simulink model "swerve_chassis"  (R2025b)
settings: Solver=VariableStepAuto  StartTime=0.0  StopTime=20  RelTol=1e-2  AbsTol=1e-3
undefined symbols (not defined in the file): X, Y, Z
libraries: sm_lib x35, nesl_utility x18, slpidlib x8
(part 2 of 2)

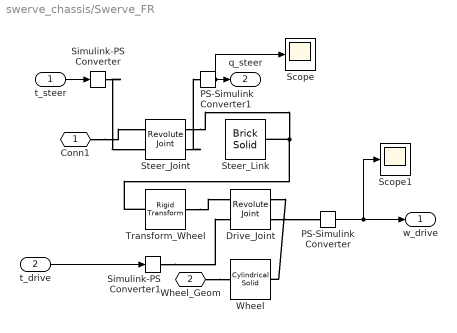
== system swerve_chassis/Swerve_FR ==
  t_steer : Inport
  t_drive : Inport  Port=2
  Drive_Joint : sm_lib/Joints/Revolute Joint  JointMode=Normal  CompositeWrenchDir=FollowerOnBase  CompositeWrenchFrame=BaseFrame  SenseConstraintForce=off  SenseConstraintTorque=off  SenseTotalForce=off  SenseTotalTorque=off  PositionTargetSpecify=off  PositionTargetPriority=High  PositionTargetValue=0  PositionTargetValueUnits=deg  VelocityTargetSpecify=off  VelocityTargetPriority=High  VelocityTargetValue=0  VelocityTargetValueUnits=deg/s  EquilibriumPosition=0  EquilibriumPositionUnits=deg  SpringStiffness=0  SpringStiffnessUnits=N*m/deg  DampingCoefficient=0  DampingCoefficientUnits=N*m/(deg/s)  LowerLimitSpecify=off  LowerLimitBound=-90  LowerLimitBoundUnits=deg  LowerLimitStiffness=1e4  LowerLimitStiffnessUnits=N*m/deg  LowerLimitDamping=10  LowerLimitDampingUnits=N*m/(deg/s)  LowerLimitTransitionRegionWidth=0.1  LowerLimitTransitionRegionWidthUnits=deg  UpperLimitSpecify=off  UpperLimitBound=90  UpperLimitBoundUnits=deg  UpperLimitStiffness=1e4  UpperLimitStiffnessUnits=N*m/deg  UpperLimitDamping=10  UpperLimitDampingUnits=N*m/(deg/s)  UpperLimitTransitionRegionWidth=0.1  UpperLimitTransitionRegionWidthUnits=deg  TorqueActuationMode=InputTorque  MotionActuationMode=ComputedMotion  SensePosition=off  SenseVelocity=on  SenseAcceleration=off  SenseTorqueForce=off  SenseLowerLimitTorqueForce=off  SenseUpperLimitTorqueForce=off
  PS-Simulink Converter : nesl_utility/PS-Simulink Converter  PhysicalDomain=network_engine_domain  SubClassName=ps_output  LeftPortType=input  RightPortType=output  PseudoPeriodic=off  Frequencies=[]  VectorFormat=inherit  Unit=rad/s  AffineConversion=off
  PS-Simulink Converter1 : nesl_utility/PS-Simulink Converter  PhysicalDomain=network_engine_domain  SubClassName=ps_output  LeftPortType=input  RightPortType=output  PseudoPeriodic=off  Frequencies=[]  VectorFormat=inherit  Unit=rad  AffineConversion=off
  Scope : Scope
      settings: ActiveDisplayYMinimum=-1  ActiveDisplayYMaximum=1  DataLoggingVariableName=ScopeData2
  Scope1 : Scope
      settings: ActiveDisplayYMinimum=-1  ActiveDisplayYMaximum=1  DataLoggingVariableName=ScopeData3
  Simulink-PS Converter : nesl_utility/Simulink-PS Converter  PhysicalDomain=network_engine_domain  SubClassName=ps_input  LeftPortType=input  RightPortType=output  PseudoPeriodic=off  Frequencies=[]  NoiseDistribution=none  NoiseParameters=[]  Unit=1  AffineConversion=off  FilteringAndDerivatives=provide  SimscapeFilterOrder=1  InputFilterTimeConstant=0.001  UdotUserProvided=0
  Simulink-PS Converter1 : nesl_utility/Simulink-PS Converter  PhysicalDomain=network_engine_domain  SubClassName=ps_input  LeftPortType=input  RightPortType=output  PseudoPeriodic=off  Frequencies=[]  NoiseDistribution=none  NoiseParameters=[]  Unit=1  AffineConversion=off  FilteringAndDerivatives=provide  SimscapeFilterOrder=1  InputFilterTimeConstant=0.001  UdotUserProvided=0
  Steer_Joint : sm_lib/Joints/Revolute Joint  JointMode=Normal  CompositeWrenchDir=FollowerOnBase  CompositeWrenchFrame=BaseFrame  SenseConstraintForce=off  SenseConstraintTorque=off  SenseTotalForce=off  SenseTotalTorque=off  PositionTargetSpecify=off  PositionTargetPriority=High  PositionTargetValue=0  PositionTargetValueUnits=deg  VelocityTargetSpecify=off  VelocityTargetPriority=High  VelocityTargetValue=0  VelocityTargetValueUnits=deg/s  EquilibriumPosition=0  EquilibriumPositionUnits=deg  SpringStiffness=0  SpringStiffnessUnits=N*m/deg  DampingCoefficient=0  DampingCoefficientUnits=N*m/(deg/s)  LowerLimitSpecify=off  LowerLimitBound=-90  LowerLimitBoundUnits=deg  LowerLimitStiffness=1e4  LowerLimitStiffnessUnits=N*m/deg  LowerLimitDamping=10  LowerLimitDampingUnits=N*m/(deg/s)  LowerLimitTransitionRegionWidth=0.1  LowerLimitTransitionRegionWidthUnits=deg  UpperLimitSpecify=off  UpperLimitBound=90  UpperLimitBoundUnits=deg  UpperLimitStiffness=1e4  UpperLimitStiffnessUnits=N*m/deg  UpperLimitDamping=10  UpperLimitDampingUnits=N*m/(deg/s)  UpperLimitTransitionRegionWidth=0.1  UpperLimitTransitionRegionWidthUnits=deg  TorqueActuationMode=InputTorque  MotionActuationMode=ComputedMotion  SensePosition=on  SenseVelocity=off  SenseAcceleration=off  SenseTorqueForce=off  SenseLowerLimitTorqueForce=off  SenseUpperLimitTorqueForce=off
  Steer_Link : sm_lib/Body Elements/Brick Solid  BrickDimensions=[0.05 0.05 0.1]  BrickDimensionsUnits=m  ExportEntireGeometry=off  InertiaType=Custom  BasedOnType=Density  Density=1000  DensityUnits=kg/m^3  Mass=1  MassUnits=kg  CenterOfMass=[0 0 0]  CenterOfMassUnits=m  MomentsOfInertia=[1 1 1]  MomentsOfInertiaUnits=kg*m^2  ProductsOfInertia=[0 0 0]  ProductsOfInertiaUnits=kg*m^2  GraphicType=FromGeometry  MarkerShape=Sphere  MarkerSize=10  GraphicVisPropType=SimpleVisualProperties  GraphicDiffuseColor=[1 1 0]  GraphicOpacity=1  GraphicSpecularColor=[0.5 0.5 0.5 1.0]  GraphicAmbientColor=[0.15 0.15 0.15 1.0]  GraphicEmissiveColor=[0.0 0.0 0.0 1.0]  GraphicShininess=75  DoExposeReferenceFrame=on  SerializedFrames=<Frames/>
  Transform_Wheel : sm_lib/Frames and Transforms/Rigid Transform  RotationMethod=StandardAxis  FollAlignAxisA=+X  BaseAlignAxisA=+Y  FollAlignAxisB=+Y  BaseAlignAxisB=+Z  RotationStandardAxis=+X  RotationAngle=90  RotationAngleUnits=deg  RotationArbitraryAxis=[0 0 1]  RotationSequenceAxes=FollowerAxes  RotationSequence=XYX  RotationSequenceAngles=[0 0 0]  RotationSequenceAnglesUnits=deg  RotationMatrix=[1 0 0;0 1 0;0 0 1]  Quaternion=[1 0 0 0]  TranslationMethod=StandardAxis  TranslationCartesianOffset=[0 0 0]  TranslationCartesianOffsetUnits=m  TranslationStandardAxis=-Z  TranslationStandardOffset=0.05  TranslationStandardOffsetUnits=m  TranslationROffset=0  TranslationROffsetUnits=m  TranslationThetaOffset=0  TranslationThetaOffsetUnits=deg  TranslationZOffset=0  TranslationZOffsetUnits=m
  Wheel : sm_lib/Body Elements/Cylindrical Solid  CylinderRadius=0.05  CylinderRadiusUnits=m  CylinderLength=0.03  CylinderLengthUnits=m  ExportEntireGeometry=on  InertiaType=Custom  BasedOnType=Density  Density=1000  DensityUnits=kg/m^3  Mass=1  MassUnits=kg  CenterOfMass=[0 0 0]  CenterOfMassUnits=m  MomentsOfInertia=[1 1 1]  MomentsOfInertiaUnits=kg*m^2  ProductsOfInertia=[0 0 0]  ProductsOfInertiaUnits=kg*m^2  GraphicType=FromGeometry  MarkerShape=Sphere  MarkerSize=10  GraphicVisPropType=AdvancedVisualProperties  GraphicDiffuseColor=[1 0 0]  GraphicOpacity=1  GraphicSpecularColor=[0.5 0.5 0.5 1.0]  GraphicAmbientColor=[0.15 0.15 0.15 1.0]  GraphicEmissiveColor=[0.0 0.0 0.0 1.0]  GraphicShininess=75  DoExposeReferenceFrame=on  SerializedFrames=<Frames/>
  Conn1 : PMIOPort  Side=Left
  Wheel_Geom : PMIOPort  Port=2  Side=Left
  w_drive : Outport
  q_steer : Outport  Port=2
  wires:
  t_steer/1 -> Simulink-PS Converter/1
  PS-Simulink Converter1/1 -> Scope/1, q_steer/1
  t_drive/1 -> Simulink-PS Converter1/1
  PS-Simulink Converter/1 -> Scope1/1, w_drive/1
  connections:
  Conn1/RConn1 -- Steer_Joint/LConn1
  Steer_Joint/RConn1 -- Transform_Wheel/LConn1 -- Steer_Link/RConn1
  Transform_Wheel/RConn1 -- Drive_Joint/LConn1
  Drive_Joint/RConn1 -- Wheel/RConn1
  Wheel_Geom/RConn1 -- Wheel/LConn1
  Simulink-PS Converter/RConn1 -- Steer_Joint/LConn2
  Simulink-PS Converter1/RConn1 -- Drive_Joint/LConn2
  Drive_Joint/RConn2 -- PS-Simulink Converter/LConn1
  Steer_Joint/RConn2 -- PS-Simulink Converter1/LConn1

== matlab function swerve_chassis/MATLAB Function1 ==
  data: vx input; FL_Angle output; FL_Vel output; vy input; omega input; FR_Angle output; FR_Vel output; BL_Angle output; BL_Vel output; BR_Angle output; BR_Vel output
function [FL_Angle, FL_Vel, FR_Angle, FR_Vel, BL_Angle, BL_Vel, BR_Angle, BR_Vel] = IK_fcn(vx, vy, omega)
    % --- 尺寸参数 ---
    L = 0.5;  % 车长 (影响 Y 轴分量)
    W = 0.5;  % 车宽 (影响 X 轴分量)
    R = 0.05; % 车轮半径 (米)
    
    % --- 1. 绝对纯净的数学速度分量 (修复了 L 和 W 的交叉对应) ---
    FL_vx = vx - omega * (W / 2);
    FL_vy = vy + omega * (L / 2);
    
    FR_vx = vx + omega * (W / 2);
    FR_vy = vy + omega * (L / 2);
    
    BL_vx = vx - omega * (W / 2);
    BL_vy = vy - omega * (L / 2);
    
    BR_vx = vx + omega * (W / 2);
    BR_vy = vy - omega * (L / 2);

    % --- 2. 角度对齐 ---
    % 因为你已经在 Simscape 硬件的三维模型里加了 180 度，这里必须是 0
    offset = 0; 
    
    FL_Angle = atan2(FL_vy, FL_vx) + offset;
    FR_Angle = atan2(FR_vy, FR_vx) + offset;
    BL_Angle = atan2(BL_vy, BL_vx) + offset;
    BR_Angle = atan2(BR_vy, BR_vx) + offset;

    % --- 3. 速度输出转换 (直接除以车轮半径 R，将 m/s 转换为 rad/s) ---
    FL_Vel = sqrt(FL_vx^2 + FL_vy^2) / R;
    BL_Vel = sqrt(BL_vx^2 + BL_vy^2) / R;
    FR_Vel = sqrt(FR_vx^2 + FR_vy^2) / R; 
    BR_Vel = sqrt(BR_vx^2 + BR_vy^2) / R; 
end

== matlab function swerve_chassis/MATLAB Function ==
  data: vx_world input; vx_robot output; vy_world input; theta input; vy_robot output
function [vx_robot, vy_robot] = fcn(vx_world, vy_world, theta)
    % 1. 保留这个反馈取反，用来压制底盘的钟摆自转（因为物理关节测量极性相反）
    theta_corrected = -theta; 
    
    % 2. 恢复最纯粹、最标准的二维正交旋转矩阵
    % (绝对不要再把 sin 和 cos 颠倒，也不要乱加负号了！)
    vx_robot =  vx_world * cos(theta_corrected) + vy_world * sin(theta_corrected);
    vy_robot = -vx_world * sin(theta_corrected) + vy_world * cos(theta_corrected);
end
